simulink model "p2_changed_vectros"  (R2021a)
settings: Solver=FixedStepAuto  StartTime=0.0  StopTime=inf  RelTol=1e-3
settings Model: CodeVerificationMode=processor-in-the-loop (pil)  EnablePacing=on  PacingRate=0.350000  Creator=Abbas  LastModifiedBy=smrh1
settings HardwareCC: ProdLongLongMode=on

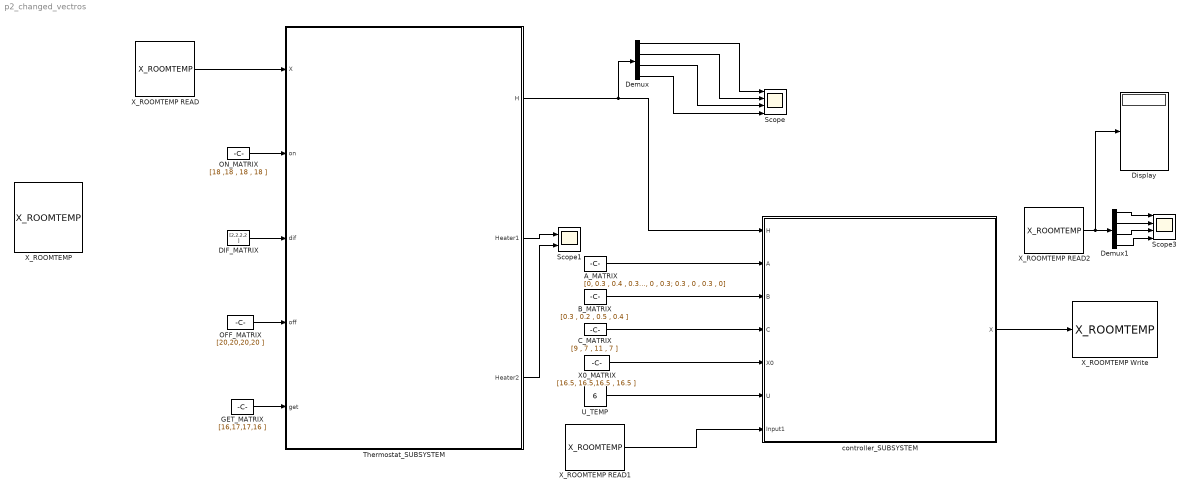
== system p2_changed_vectros ==
  A_MATRIX : Constant  Value=[0, 0.3 , 0.4 , 0.3 ; 0.3 , 0 , 0.5 , 0 ; 0.4 , 0.5 , 0 , 0.3; 0.3 , 0 , 0.3 , 0]
  B_MATRIX : Constant  Value=[0.3 , 0.2 , 0.5 , 0.4 ]
  C_MATRIX : Constant  Value=[9 , 7 , 11 , 7 ]
  DIF_MATRIX : Constant  Value=[2,2,2,2 ]
  Demux : Demux
  Demux1 : Demux
  Display : Display
  GET_MATRIX : Constant  Value=[16,17,17,16 ]
  OFF_MATRIX : Constant  Value=[20,20,20,20 ]
  ON_MATRIX : Constant  Value=[18 ,18 , 18 , 18 ]
  Scope : Scope  NumInputPorts=4
  Scope1 : Scope  NumInputPorts=2
  Scope3 : Scope  NumInputPorts=4
  Thermostat_SUBSYSTEM : Subsystem
  U_TEMP : Constant  Value=6
  X0_MATRIX : Constant  Value=[16.5, 16.5,16.5 , 16.5 ]
  X_ROOMTEMP : DataStoreMemory  DataStoreName=X_ROOMTEMP  ReadBeforeWriteMsg=warning  WriteAfterWriteMsg=warning  WriteAfterReadMsg=warning  InitialValue=[16.5,16.5,16.5,16.5]  ShowAdditionalParam=off
  X_ROOMTEMP READ : DataStoreRead  DataStoreName=X_ROOMTEMP  IndexOptions=Index vector (dialog)  Indices=1  OutputSizes=1
  X_ROOMTEMP READ1 : DataStoreRead  DataStoreName=X_ROOMTEMP  IndexOptions=Index vector (dialog)  Indices=1  OutputSizes=1
  X_ROOMTEMP READ2 : DataStoreRead  DataStoreName=X_ROOMTEMP  IndexOptions=Index vector (dialog)  Indices=1  OutputSizes=1
  X_ROOMTEMP Write : DataStoreWrite  DataStoreName=X_ROOMTEMP  IndexOptions=Index vector (dialog)  Indices=1  OutputSizes=1
  controller_SUBSYSTEM : Subsystem
  wires:
  Thermostat_SUBSYSTEM/1(H) -> Demux/1, controller_SUBSYSTEM/1(H)
  controller_SUBSYSTEM/1(X) -> X_ROOMTEMP Write/1
  X_ROOMTEMP READ/1 -> Thermostat_SUBSYSTEM/1(X)
  A_MATRIX/1 -> controller_SUBSYSTEM/2(A)
  B_MATRIX/1 -> controller_SUBSYSTEM/3(B)
  C_MATRIX/1 -> controller_SUBSYSTEM/4(C)
  X0_MATRIX/1 -> controller_SUBSYSTEM/5(X0)
  DIF_MATRIX/1 -> Thermostat_SUBSYSTEM/3(dif)
  GET_MATRIX/1 -> Thermostat_SUBSYSTEM/5(get)
  OFF_MATRIX/1 -> Thermostat_SUBSYSTEM/4(off)
  ON_MATRIX/1 -> Thermostat_SUBSYSTEM/2(on)
  U_TEMP/1 -> controller_SUBSYSTEM/6(U)
  X_ROOMTEMP READ1/1 -> controller_SUBSYSTEM/7(Input1)
  Thermostat_SUBSYSTEM/2(Heater1) -> Scope1/1
  Thermostat_SUBSYSTEM/3(Heater2) -> Scope1/2
  Demux/1 -> Scope/1
  Demux/2 -> Scope/2
  Demux/3 -> Scope/3
  Demux/4 -> Scope/4
  Demux1/1 -> Scope3/1
  Demux1/2 -> Scope3/2
  Demux1/3 -> Scope3/3
  Demux1/4 -> Scope3/4
  X_ROOMTEMP READ2/1 -> Display/1, Demux1/1

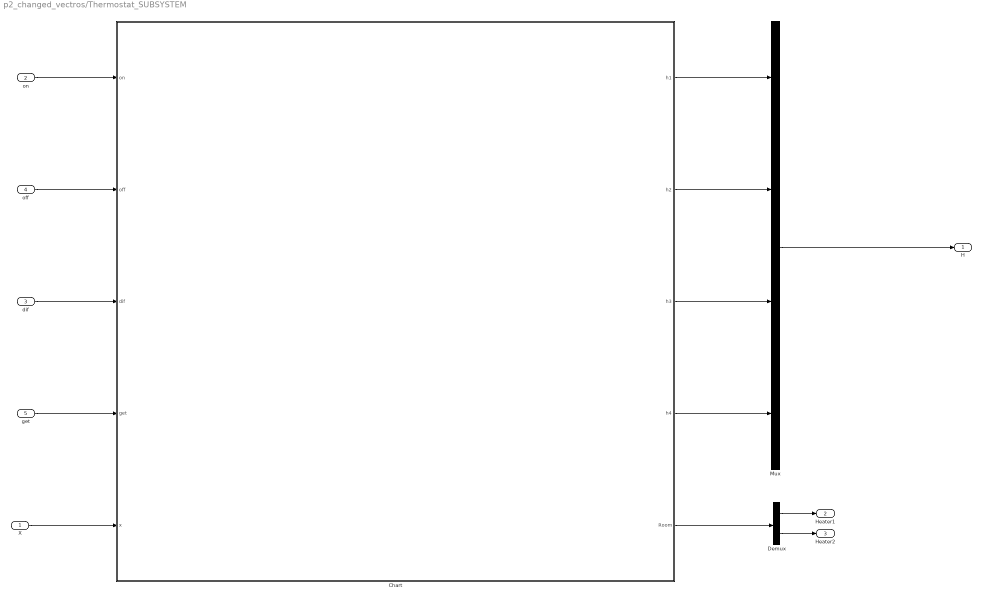
== system p2_changed_vectros/Thermostat_SUBSYSTEM ==
  X : Inport
  on : Inport  Port=2
  dif : Inport  Port=3
  off : Inport  Port=4
  get : Inport  Port=5
  Chart : Stateflow chart  TreatAsAtomicUnit=on
  Demux : Demux  Outputs=2
  Mux : Mux
  H : Outport
  Heater1 : Outport  Port=2
  Heater2 : Outport  Port=3
  wires:
  Chart/1(h1) -> Mux/1
  Chart/2(h2) -> Mux/2
  Chart/3(h3) -> Mux/3
  Chart/4(h4) -> Mux/4
  X/1 -> Chart/5(x)
  off/1 -> Chart/2(off)
  on/1 -> Chart/1(on)
  dif/1 -> Chart/3(dif)
  get/1 -> Chart/4(get)
  Mux/1 -> H/1
  Chart/5(Room) -> Demux/1
  Demux/1 -> Heater1/1
  Demux/2 -> Heater2/1

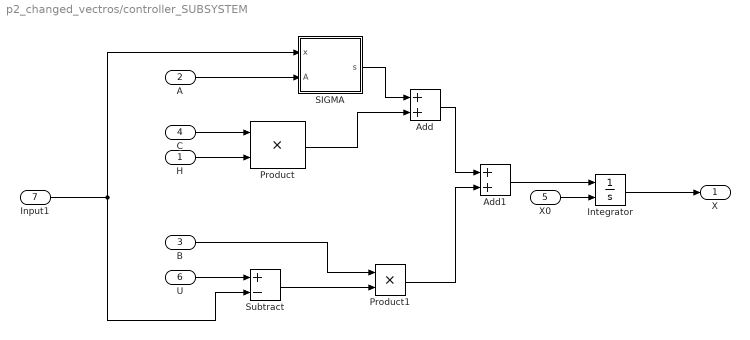
== system p2_changed_vectros/controller_SUBSYSTEM ==
  H : Inport
  A : Inport  Port=2
  B : Inport  Port=3
  C : Inport  Port=4
  X0 : Inport  Port=5
  U : Inport  Port=6
  Input1 : Inport  Port=7
  Add : Sum
  Add1 : Sum
  Integrator : Integrator  InitialConditionSource=external
  Product : Product
  Product1 : Product
  SIGMA : Stateflow chart  TreatAsAtomicUnit=on
  Subtract : Sum  Inputs=+-
  X : Outport
  wires:
  C/1 -> Product/1
  H/1 -> Product/2
  U/1 -> Subtract/1
  B/1 -> Product1/1
  Subtract/1 -> Product1/2
  A/1 -> SIGMA/2(A)
  Product/1 -> Add/2
  SIGMA/1(s) -> Add/1
  Product1/1 -> Add1/2
  Add/1 -> Add1/1
  Add1/1 -> Integrator/1
  X0/1 -> Integrator/2
  Integrator/1 -> X/1
  Input1/1 -> SIGMA/1(x), Subtract/2

== stateflow chart p2_changed_vectros/Thermostat_SUBSYSTEM/Chart ==
  state st13
    entry:
    h2 = 0;
    h4 = 0;
    Room=[1,3];
    state s1 [parallel]
      settings: executionOrder=1
      state s1_on
        entry:
        h1 = 1
      state s1_off
        entry:
        h1 = 0
      (default) -> st13.s1.s1_on
      st13.s1.s1_on -> st13.s1.s1_off : [x(1)>=off(1)]
      st13.s1.s1_off -> st13.s1.s1_on : [x(1)<=on(1)]
    state s3 [parallel]
      settings: executionOrder=2
      state s3_on
        entry:
        h3 = 1
      state s3_off
        entry:
        h3 = 0
      (default) -> st13.s3.s3_on
      st13.s3.s3_on -> st13.s3.s3_off : [x(3)>=off(3)]
      st13.s3.s3_off -> st13.s3.s3_on : [x(3)<=on(3)]
  state st14
    entry:
    h2 = 0;
    h3 = 0;
    Room=[1,4];
    state s1 [parallel]
      settings: executionOrder=1
      state s1_on
        entry:
        h1 = 1
      state s1_off
        entry:
        h1 = 0
      (default) -> st14.s1.s1_on
      st14.s1.s1_on -> st14.s1.s1_off : [x(1)>=off(1)]
      st14.s1.s1_off -> st14.s1.s1_on : [x(1)<=on(1)]
    state s4 [parallel]
      settings: executionOrder=2
      state s4_on
        entry:
        h4 = 1
      state s4_off
        entry:
        h4 = 0
      (default) -> st14.s4.s4_on
      st14.s4.s4_on -> st14.s4.s4_off : [x(4)>=off(4)]
      st14.s4.s4_off -> st14.s4.s4_on : [x(4)<=on(4)]
  state st12
    entry:
    h3 = 0;
    h4 = 0;
    Room=[1,2];
    state s1 [parallel]
      settings: executionOrder=1
      state s1_on1
        entry:
        h1 = 1
      state s1_off
        entry:
        h1 = 0
      (default) -> s1_on1
      s1_on1 -> st12.s1.s1_off : [x(1)>=off(1) ]
      st12.s1.s1_off -> s1_on1 : [x(1)<=on(1) ]
    state s2 [parallel]
      settings: executionOrder=2
      state s2_on
        entry:
        h2 = 1
      state s1_off1
        entry:
        h2 = 0
      (default) -> st12.s2.s2_on
      st12.s2.s2_on -> s1_off1 : [x(2)>=off(2)]
      s1_off1 -> st12.s2.s2_on : [x(2)<=on(2)]
  state st24
    entry:
    h1 = 0;
    h3 = 0;
    Room=[1,3];
    state s2 [parallel]
      settings: executionOrder=1
      state s2_on
        entry:
        h2 = 1
      state s2_off
        entry:
        h2 = 0
      (default) -> st24.s2.s2_on
      st24.s2.s2_on -> s2_off : [x(2)>=off(2)]
      s2_off -> st24.s2.s2_on : [x(2)<=on(2)]
    state s4 [parallel]
      settings: executionOrder=2
      state s4_on
        entry:
        h4 = 1
      state s4_off
        entry:
        h4 = 0
      (default) -> st24.s4.s4_on
      st24.s4.s4_on -> st24.s4.s4_off : [x(4)>=off(4)]
      st24.s4.s4_off -> st24.s4.s4_on : [x(4)<=on(4)]
  state st34
    entry:
    h1 = 0;
    h2 = 0;
    Room=[3,4];
    state s3 [parallel]
      settings: executionOrder=1
      state s3_on
        entry:
        h3 = 1
      state s3_off
        entry:
        h3 = 0
      (default) -> st34.s3.s3_on
      st34.s3.s3_on -> st34.s3.s3_off : [x(3)>=off(3)]
      st34.s3.s3_off -> st34.s3.s3_on : [x(3)<=on(3)]
    state s4 [parallel]
      settings: executionOrder=2
      state s4_on
        entry:
        h4 = 1
      state s4_off
        entry:
        h4 = 0
      (default) -> st34.s4.s4_on
      st34.s4.s4_on -> st34.s4.s4_off : [x(4)>=off(4)]
      st34.s4.s4_off -> st34.s4.s4_on : [x(4)<=on(4)]
  state st23
    entry:
    h1 = 0;
    h4 = 0;
    Room=[2,3];
    state s2 [parallel]
      settings: executionOrder=1
      state s2_on
        entry:
        h2 = 1;
      state s1_off
        entry:
        h2 = 0;
      (default) -> st23.s2.s2_on
      st23.s2.s2_on -> st23.s2.s1_off : [x(2)>= off(2)]
      st23.s2.s1_off -> st23.s2.s2_on : [x(2)<=on(2)]
    state s3 [parallel]
      settings: executionOrder=2
      state s3_on
        entry:
        h3 = 1;
      state s3_off
        entry:
        h3 = 0;
      (default) -> st23.s3.s3_on
      st23.s3.s3_on -> st23.s3.s3_off : [x(3)>=off(3)]
      st23.s3.s3_off -> st23.s3.s3_on : [x(3)<=on(3) ]
  state start
    entry:
    h1=0
    h4=0
    h2=1;
    h3=1;
    Room=[2,3]
  st13 -> st14 [order 2] : [x(3)-x(4)>=dif(4) & x(4)<=get(4)]{h1=0;h3=0}
  st12 -> st13 [order 1] : [x(2)-x(3)>=dif(3) & x(3)<=get(3)]{h1=0;h2=0;}
  st13 -> st12 [order 1] : [x(3)-x(2)>=dif(2) & x(2)<=get(2)]{h1=0;h3=0;}
  st14 -> st13 [order 1] : [x(4)-x(3)>=dif(3) & x(3)<=get(3)]{h1=0;h4=0;}
  st13 -> st23 [order 3] : [(x(1)-x(2)>=dif(2) & x(2)<=get(2))]{h1=0;h3=0;}
  st13 -> st34 [order 4] : [x(1)-x(4)>=dif(4) & x(4)<=get(4)]{h1=0;h3=0;}
  st23 -> st13 [order 2] : [(x(2)-x(1)>=dif(1) & x(1)<=get(1))]{h2=0;h3=0}
  st34 -> st13 [order 1] : [x(4)-x(1)>=dif(1) & x(1)<=get(1)]{h3=0;h4=0;}
  st12 -> st14 [order 3] : [x(2)-x(4)>=dif(4) & x(4)<=get(4)]{h1=0;h2=0;}
  st14 -> st12 [order 2] : [x(4)-x(2)>=dif(2) & x(2)<=get(2)]{h1=0;h4=0;}
  st14 -> st24 [order 3] : [x(4)-x(2)>=dif(2) & x(2)<=get(2)]{h1=0;h4=0;}
  st24 -> st14 [order 2] : [x(2)-x(4)>=dif(4) & x(4)<=get(4)]{h2=0;h4=0;}
  st14 -> st34 [order 4] : [x(1)-x(3)>=dif(3) & x(3)<=get(3)]{h1=0;h4=0;}
  st34 -> st14 [order 2] : [x(3)-x(1)>=dif(1) & x(1)<=get(1)]{h3=0;h4=0;}
  st12 -> st23 [order 2] : [x(1)-x(3)>=dif(3) & x(3)<=get(3)]{h1=0;h2=0;}
  st23 -> st12 [order 1] : [x(3)-x(1)>=dif(1) & x(1)<=get(1)]{h2=0;h3=0;}
  st24 -> st12 [order 1] : [x(4)-x(1)>=dif(1) & x(1)<=get(1)]{h2=0;h4=0;}
  st12 -> st24 [order 4] : [x(1)-x(4)>=dif(4) & x(4)<=get(4)]{h1=0;h2=0;}
  (default) -> start
  start -> st23
  st23 -> st24 [order 3] : [x(3)-x(4)>=dif(4) & x(4)<=get(4)]{h2=0;h3=0;}
  st24 -> st34 [order 4] : [x(2)-x(3)>=dif(3) & x(3)<=get(3)]{h2=0;h4=0;}
  st24 -> st23 [order 3] : [x(4)-x(3)>=dif(3) & x(3)<=get(3)]{h2=0;h4=0;}
  st34 -> st24 [order 4] : [x(3)-x(2)>=dif(2) & x(2)<=get(2)]{h3=0;h4=0;}
  st23 -> st34 [order 4] : [x(2)-x(4)>=dif(4) & x(4)<=get(4)]{h3=0;h2=0;}
  st34 -> st23 [order 3] : [x(4)-x(2)>=dif(2) & x(2)<=get(2)]{h3=0;h4=0;}
  data: h1 output double; h2 output double; h3 output double; h4 output double; on input; off input; dif input; get input; x input double; Room output

== stateflow chart p2_changed_vectros/controller_SUBSYSTEM/SIGMA ==
  state s3
    du:
    s(1) = A(1,2)*(x(2)-x(1)) + A(1,3)*(x(3)-x(1)) + A(1,4)*(x(4)-x(1));
    s(2) = A(2,1)*(x(1)-x(2)) + A(2,3)*(x(3)-x(2)) + A(2,4)*(x(4)-x(2));
    s(3) = A(3,1)*(x(1)-x(3)) + A(3,2)*(x(2)-x(3)) + A(3,4)*(x(4)-x(3));
    s(4) = A(4,1)*(x(1)-x(4)) + A(4,2)*(x(2)-x(4)) + A(4,3)*(x(3)-x(4));
  (default) -> s3 : {s=[0,0,0,0];}
  data: x input; A input; s output
